simulink model "Narx1Model1"  (R2017a)
settings: Solver=VariableStepAuto  StartTime=0.0  StopTime=500  RelTol=1e-3
settings Model: Creator=Korisnik  LastModifiedBy=Korisnik

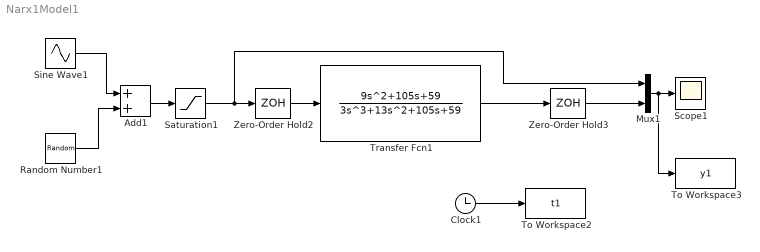
== system Narx1Model1 ==
  Add1 : Sum
  Clock1 : Clock
  Mux1 : Mux  Inputs=2
  Random Number1 : RandomNumber  Variance=0.1  SampleTime=0.1
  Saturation1 : Saturate  UpperLimit=5  LowerLimit=-5
  Scope1 : Scope
  Sine Wave1 : Sin  Amplitude=4  Frequency=0.025  SampleTime=0.1
  To Workspace2 : ToWorkspace  VariableName=t1  SaveFormat=Timeseries  SampleTime=-1
  To Workspace3 : ToWorkspace  VariableName=y1  SampleTime=-1
  Transfer Fcn1 : TransferFcn  Numerator=[0 9 105 59]  Denominator=[3 13 105 59]
  Zero-Order Hold2 : ZeroOrderHold  SampleTime=0.1
  Zero-Order Hold3 : ZeroOrderHold  SampleTime=0.1
  wires:
  Sine Wave1/1 -> Add1/1
  Random Number1/1 -> Add1/2
  Add1/1 -> Saturation1/1
  Saturation1/1 -> Mux1/1, Zero-Order Hold2/1
  Zero-Order Hold2/1 -> Transfer Fcn1/1
  Transfer Fcn1/1 -> Zero-Order Hold3/1
  Zero-Order Hold3/1 -> Mux1/2
  Mux1/1 -> To Workspace3/1, Scope1/1
  Clock1/1 -> To Workspace2/1
